simulink library "Mako_TimeScaling"  (R2024b)
settings: Solver=VariableStepAuto  StartTime=0.0  StopTime=10.0  RelTol=1e-3
settings Model: Creator=pinto  LastModifiedBy=pinto

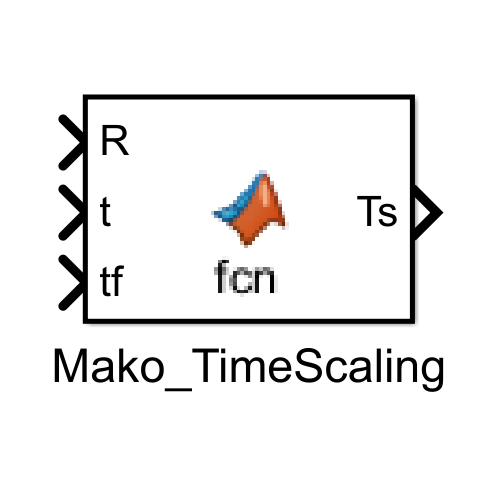
[thumbnail: Simulink's stored preview of the top-level diagram]
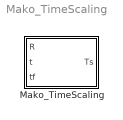
== system Mako_TimeScaling ==
  Mako_TimeScaling : MATLAB Function  TreatAsAtomicUnit=on

== matlab function Mako_TimeScaling/Mako_TimeScaling ==
  data: R input; Ts output; t input; tf input
function Ts = Mako_TimeScaling(R,t,tf)
%#codegen

%    This function was generated by the Symbolic Math Toolbox version 24.2.
%    11-Jun-2025 19:47:13

% R = complex(R);  % if required to enforce complex operations
% t = complex(t);  % if required to enforce complex operations
% tf = complex(tf);  % if required to enforce complex operations
Ts = R.*t.^2.*1.0./tf.^2.*2.013716694115407e+1-R.*t.^3.*1.0./tf.^3.*1.342477796076938e+1;
end
